simulink model "six_plus_six_AcmsteeringV09_main"  (R2014a)
settings: Solver=FixedStepDiscrete  StartTime=0.0  StopTime=10.0  FixedStep=0.0005  RelTol=1e-3
InitFcn:
  | Veh_Par_wxt
values from neighbouring files (symbols this model uses):
  acc_spdctl = [0 100]    [Veh_Par_wxt.m]
  ag_thr = ecucoder_cal(ag_thr)    [Veh_Par_wxt.m]
  B = 1.8    [Veh_Par_wxt.m]
  bra_em = 100    [Veh_Par_wxt.m]
  bra_pre_gz2 = 100/3    (= 33.3333333333)    [Veh_Par_wxt.m]
  bra_pre_gz34 = 10/3    (= 3.33333333333)    [Veh_Par_wxt.m]
  bra_pre_yd = 10/2    (= 5)    [Veh_Par_wxt.m]
  brakepre_dem_data = [0 1 2 3 4 5 6 7 8 9 10]    [Veh_Par_wxt.m]
  brakeTrq_dem_data = [0 125 251 376 502 627 753 878 1004 1129 1255]    [Veh_Par_wxt.m]
  bratrq_max = 4*1255    (= 5020)    [Veh_Par_wxt.m]
  eff_tran = 0.9    [Veh_Par_wxt.m]
  ESP_switch = ecucoder_cal(ESP_switch)    [Veh_Par_wxt.m]
  G = Mass*g    (= 15696)    [Veh_Par_wxt.m]
  kd1 = ecucoder_cal(kd1)    [Veh_Par_wxt.m]
  kd2 = 0    [Veh_Par_wxt.m]
  ki1 = ecucoder_cal(ki1)    [Veh_Par_wxt.m]
  ki2 = 1    [Veh_Par_wxt.m]
  kp1 = ecucoder_cal(kp1)    [Veh_Par_wxt.m]
  kp2 = 300    [Veh_Par_wxt.m]
  L = L1+L2    (= 2.9)    [Veh_Par_wxt.m]
  premax = 100    [Veh_Par_wxt.m]
  Radius = 0.4572/2    (= 0.2286)    [Veh_Par_wxt.m]
  RC_switch = ecucoder_cal(RC_switch)    [Veh_Par_wxt.m]
  s_opt_yi = 0.15    [Veh_Par_wxt.m]
  s_opt_zhuan = 0.8    [Veh_Par_wxt.m]
  s_opt_zhuan_add = 0.05    [Veh_Par_wxt.m]
  s_opt_zhuan_table = [0.8 0.8 0.3 0.3]    [Veh_Par_wxt.m]
  spd_map_mot = [0 499.85 999.79 1500 2000 2500 3000 3500 4000 4500 4999.8 5999.8]    [Veh_Par_wxt.m]
  spd_spdctl = [0 500]    [Veh_Par_wxt.m]
  speed_thr_park = 5/3.6/Radius*tras_ratio*30/pi    (= 464.143899364)    [Veh_Par_wxt.m]
  TCS_switch = ecucoder_cal(TCS_switch)    [Veh_Par_wxt.m]
  tras_ratio = 8    [Veh_Par_wxt.m]
  trq_map_mot = [70.5 70.012 71.154 65.797 53.917 45.159 38.073 32.685 27.48 17.133 14.949 10.07]    [Veh_Par_wxt.m]
  trqmax_yd = 70.5    [Veh_Par_wxt.m]
  trqmax_zx = 70.5    [Veh_Par_wxt.m]
  trqmaxneg = -70.5    [Veh_Par_wxt.m]
  v_gain = 0.9    [Veh_Par_wxt.m]
  v_table = [0 5 20 100]    [Veh_Par_wxt.m]
  v_thr_park = 5    [Veh_Par_wxt.m]
  zhidong_bianmazhi = [-140000 750000]    [Veh_Par_wxt.m]
  zhidong_down = -140000    [Veh_Par_wxt.m]
  zhidong_up = 750000    [Veh_Par_wxt.m]
  zhidong_youmen = [0 100]    [Veh_Par_wxt.m]
  zhuanxiang_bianmazhi = [-400000 0 400000]    [Veh_Par_wxt.m]
  zhuanxiang_down = -400000    [Veh_Par_wxt.m]
  zhuanxiang_up = 400000    [Veh_Par_wxt.m]
  zhuanxiang_youmen = [-100 0 100]    [Veh_Par_wxt.m]
undefined symbols (not defined in the file or in its folder): ecucoder_acal, guzhang_lf, guzhang_lm, guzhang_lr, guzhang_rf, guzhang_rm, guzhang_rr, myFIS
libraries: simulink x979, ec5744lib x59, fuzblock x2
(part 9 of 26)

== system six_plus_six_AcmsteeringV09_main/Data_input/MCU1_3/MCU1 ==
  input : Inport
  Enable : EnablePort
  Demux : Demux  Outputs=8
  MCU1_ControlTemp_Ad : Sum
  MCU1_ControlTemp_Convert : DataTypeConversion  OutDataTypeStr=uint32
  MCU1_ControlTemp_F : Gain
  MCU1_ControlTemp_L : simulink/Logic and Bit Operations/Bitwise Operator  logicop=AND  UseBitMask=on  BitMask=255  BitMaskRealWorld=Stored Integer
  MCU1_ControlTemp_O : Constant  Value=-40  OutDataTypeStr=single
  MCU1_ControlTemp_S : ArithShift
  MCU1_ControlTemp_Sub : Subsystem
  MCU1_ControlTemp_sat : Saturate  UpperLimit=215  LowerLimit=-40
  MCU1_ControlTempcv : DataTypeConversion
  MCU1_Idc_Ad : Sum
  MCU1_Idc_Convert : DataTypeConversion  OutDataTypeStr=uint32
  MCU1_Idc_F : Gain  Gain=0.1
  MCU1_Idc_L : simulink/Logic and Bit Operations/Bitwise Operator  logicop=AND  UseBitMask=on  BitMask=65535  BitMaskRealWorld=Stored Integer
  MCU1_Idc_O : Constant  Value=-1600  OutDataTypeStr=single
  MCU1_Idc_S : ArithShift
  MCU1_Idc_Sub : Subsystem
  MCU1_Idc_sat : Saturate  UpperLimit=1600  LowerLimit=-1600
  MCU1_Idccv : DataTypeConversion
  MCU1_Idcinput3_Ad : Sum
  MCU1_Idcinput3_C : Constant  Value=256
  MCU1_Idcinput3_P : Product
  MCU1_MotorTemp_Ad : Sum
  MCU1_MotorTemp_Convert : DataTypeConversion  OutDataTypeStr=uint32
  MCU1_MotorTemp_F : Gain
  MCU1_MotorTemp_L : simulink/Logic and Bit Operations/Bitwise Operator  logicop=AND  UseBitMask=on  BitMask=255  BitMaskRealWorld=Stored Integer
  MCU1_MotorTemp_O : Constant  Value=-40  OutDataTypeStr=single
  MCU1_MotorTemp_S : ArithShift
  MCU1_MotorTemp_Sub : Subsystem
  MCU1_MotorTemp_sat : Saturate  UpperLimit=215  LowerLimit=-40
  MCU1_MotorTempcv : DataTypeConversion
  MCU1_PowerFdk_Ad : Sum
  MCU1_PowerFdk_Convert : DataTypeConversion  OutDataTypeStr=uint32
  MCU1_PowerFdk_F : Gain
  MCU1_PowerFdk_L : simulink/Logic and Bit Operations/Bitwise Operator  logicop=AND  UseBitMask=on  BitMask=65535  BitMaskRealWorld=Stored Integer
  MCU1_PowerFdk_O : Constant  Value=0  OutDataTypeStr=single
  MCU1_PowerFdk_S : ArithShift
  MCU1_PowerFdk_Sub : Subsystem
  MCU1_PowerFdk_sat : Saturate  UpperLimit=65535  LowerLimit=0
  MCU1_PowerFdkcv : DataTypeConversion
  MCU1_PowerFdkinput5_Ad : Sum
  MCU1_PowerFdkinput5_C : Constant  Value=256
  MCU1_PowerFdkinput5_P : Product
  MCU1_Udc_Ad : Sum
  MCU1_Udc_Convert : DataTypeConversion  OutDataTypeStr=uint32
  MCU1_Udc_F : Gain  Gain=0.1
  MCU1_Udc_L : simulink/Logic and Bit Operations/Bitwise Operator  logicop=AND  UseBitMask=on  BitMask=65535  BitMaskRealWorld=Stored Integer
  MCU1_Udc_O : Constant  Value=0  OutDataTypeStr=single
  MCU1_Udc_S : ArithShift
  MCU1_Udc_Sub : Subsystem
  MCU1_Udc_sat : Saturate  UpperLimit=1000  LowerLimit=0
  MCU1_Udccv : DataTypeConversion
  MCU1_Udcinput1_Ad : Sum
  MCU1_Udcinput1_C : Constant  Value=256
  MCU1_Udcinput1_P : Product
  MCU1_ControlTemp_Out : Outport
  MCU1_MotorTemp_Out : Outport  Port=2
  MCU1_PowerFdk_Out : Outport  Port=3
  MCU1_Idc_Out : Outport  Port=4
  MCU1_Udc_Out : Outport  Port=5
  wires:
  MCU1_ControlTemp_F/1 -> MCU1_ControlTemp_Ad/1
  MCU1_ControlTemp_O/1 -> MCU1_ControlTemp_Ad/2
  MCU1_ControlTemp_Ad/1 -> MCU1_ControlTemp_sat/1
  MCU1_ControlTemp_sat/1 -> MCU1_ControlTemp_Out/1
  Demux/8 -> MCU1_ControlTemp_Sub/1(In1)
  MCU1_ControlTemp_Sub/1(Out1) -> MCU1_ControlTemp_Convert/1
  MCU1_ControlTemp_Convert/1 -> MCU1_ControlTemp_L/1
  MCU1_ControlTemp_L/1 -> MCU1_ControlTemp_S/1
  MCU1_ControlTemp_S/1 -> MCU1_ControlTempcv/1
  MCU1_ControlTempcv/1 -> MCU1_ControlTemp_F/1
  MCU1_MotorTemp_F/1 -> MCU1_MotorTemp_Ad/1
  MCU1_MotorTemp_O/1 -> MCU1_MotorTemp_Ad/2
  MCU1_MotorTemp_Ad/1 -> MCU1_MotorTemp_sat/1
  MCU1_MotorTemp_sat/1 -> MCU1_MotorTemp_Out/1
  Demux/7 -> MCU1_MotorTemp_Sub/1(In1)
  MCU1_MotorTemp_Sub/1(Out1) -> MCU1_MotorTemp_Convert/1
  MCU1_MotorTemp_Convert/1 -> MCU1_MotorTemp_L/1
  MCU1_MotorTemp_L/1 -> MCU1_MotorTemp_S/1
  MCU1_MotorTemp_S/1 -> MCU1_MotorTempcv/1
  MCU1_MotorTempcv/1 -> MCU1_MotorTemp_F/1
  MCU1_PowerFdk_F/1 -> MCU1_PowerFdk_Ad/1
  MCU1_PowerFdk_O/1 -> MCU1_PowerFdk_Ad/2
  MCU1_PowerFdk_Ad/1 -> MCU1_PowerFdk_sat/1
  MCU1_PowerFdk_sat/1 -> MCU1_PowerFdk_Out/1
  Demux/5 -> MCU1_PowerFdkinput5_P/1
  MCU1_PowerFdkinput5_C/1 -> MCU1_PowerFdkinput5_P/2
  MCU1_PowerFdkinput5_P/1 -> MCU1_PowerFdkinput5_Ad/1
  Demux/6 -> MCU1_PowerFdkinput5_Ad/2
  MCU1_PowerFdkinput5_Ad/1 -> MCU1_PowerFdk_Sub/1(In1)
  MCU1_PowerFdk_Sub/1(Out1) -> MCU1_PowerFdk_Convert/1
  MCU1_PowerFdk_Convert/1 -> MCU1_PowerFdk_L/1
  MCU1_PowerFdk_L/1 -> MCU1_PowerFdk_S/1
  MCU1_PowerFdk_S/1 -> MCU1_PowerFdkcv/1
  MCU1_PowerFdkcv/1 -> MCU1_PowerFdk_F/1
  MCU1_Idc_F/1 -> MCU1_Idc_Ad/1
  MCU1_Idc_O/1 -> MCU1_Idc_Ad/2
  MCU1_Idc_Ad/1 -> MCU1_Idc_sat/1
  MCU1_Idc_sat/1 -> MCU1_Idc_Out/1
  Demux/3 -> MCU1_Idcinput3_P/1
  MCU1_Idcinput3_C/1 -> MCU1_Idcinput3_P/2
  MCU1_Idcinput3_P/1 -> MCU1_Idcinput3_Ad/1
  Demux/4 -> MCU1_Idcinput3_Ad/2
  MCU1_Idcinput3_Ad/1 -> MCU1_Idc_Sub/1(In1)
  MCU1_Idc_Sub/1(Out1) -> MCU1_Idc_Convert/1
  MCU1_Idc_Convert/1 -> MCU1_Idc_L/1
  MCU1_Idc_L/1 -> MCU1_Idc_S/1
  MCU1_Idc_S/1 -> MCU1_Idccv/1
  MCU1_Idccv/1 -> MCU1_Idc_F/1
  MCU1_Udc_F/1 -> MCU1_Udc_Ad/1
  MCU1_Udc_O/1 -> MCU1_Udc_Ad/2
  MCU1_Udc_Ad/1 -> MCU1_Udc_sat/1
  MCU1_Udc_sat/1 -> MCU1_Udc_Out/1
  Demux/1 -> MCU1_Udcinput1_P/1
  MCU1_Udcinput1_C/1 -> MCU1_Udcinput1_P/2
  MCU1_Udcinput1_P/1 -> MCU1_Udcinput1_Ad/1
  Demux/2 -> MCU1_Udcinput1_Ad/2
  MCU1_Udcinput1_Ad/1 -> MCU1_Udc_Sub/1(In1)
  MCU1_Udc_Sub/1(Out1) -> MCU1_Udc_Convert/1
  MCU1_Udc_Convert/1 -> MCU1_Udc_L/1
  MCU1_Udc_L/1 -> MCU1_Udc_S/1
  MCU1_Udc_S/1 -> MCU1_Udccv/1
  MCU1_Udccv/1 -> MCU1_Udc_F/1
  input/1 -> Demux/1

== system six_plus_six_AcmsteeringV09_main/Data_input/MCU1_4/MCU1 ==
  input : Inport
  Enable : EnablePort
  Demux : Demux  Outputs=8
  MCU1_ControlTemp_Ad : Sum
  MCU1_ControlTemp_Convert : DataTypeConversion  OutDataTypeStr=uint32
  MCU1_ControlTemp_F : Gain
  MCU1_ControlTemp_L : simulink/Logic and Bit Operations/Bitwise Operator  logicop=AND  UseBitMask=on  BitMask=255  BitMaskRealWorld=Stored Integer
  MCU1_ControlTemp_O : Constant  Value=-40  OutDataTypeStr=single
  MCU1_ControlTemp_S : ArithShift
  MCU1_ControlTemp_Sub : Subsystem
  MCU1_ControlTemp_sat : Saturate  UpperLimit=215  LowerLimit=-40
  MCU1_ControlTempcv : DataTypeConversion
  MCU1_Idc_Ad : Sum
  MCU1_Idc_Convert : DataTypeConversion  OutDataTypeStr=uint32
  MCU1_Idc_F : Gain  Gain=0.1
  MCU1_Idc_L : simulink/Logic and Bit Operations/Bitwise Operator  logicop=AND  UseBitMask=on  BitMask=65535  BitMaskRealWorld=Stored Integer
  MCU1_Idc_O : Constant  Value=-1600  OutDataTypeStr=single
  MCU1_Idc_S : ArithShift
  MCU1_Idc_Sub : Subsystem
  MCU1_Idc_sat : Saturate  UpperLimit=1600  LowerLimit=-1600
  MCU1_Idccv : DataTypeConversion
  MCU1_Idcinput3_Ad : Sum
  MCU1_Idcinput3_C : Constant  Value=256
  MCU1_Idcinput3_P : Product
  MCU1_MotorTemp_Ad : Sum
  MCU1_MotorTemp_Convert : DataTypeConversion  OutDataTypeStr=uint32
  MCU1_MotorTemp_F : Gain
  MCU1_MotorTemp_L : simulink/Logic and Bit Operations/Bitwise Operator  logicop=AND  UseBitMask=on  BitMask=255  BitMaskRealWorld=Stored Integer
  MCU1_MotorTemp_O : Constant  Value=-40  OutDataTypeStr=single
  MCU1_MotorTemp_S : ArithShift
  MCU1_MotorTemp_Sub : Subsystem
  MCU1_MotorTemp_sat : Saturate  UpperLimit=215  LowerLimit=-40
  MCU1_MotorTempcv : DataTypeConversion
  MCU1_PowerFdk_Ad : Sum
  MCU1_PowerFdk_Convert : DataTypeConversion  OutDataTypeStr=uint32
  MCU1_PowerFdk_F : Gain
  MCU1_PowerFdk_L : simulink/Logic and Bit Operations/Bitwise Operator  logicop=AND  UseBitMask=on  BitMask=65535  BitMaskRealWorld=Stored Integer
  MCU1_PowerFdk_O : Constant  Value=0  OutDataTypeStr=single
  MCU1_PowerFdk_S : ArithShift
  MCU1_PowerFdk_Sub : Subsystem
  MCU1_PowerFdk_sat : Saturate  UpperLimit=65535  LowerLimit=0
  MCU1_PowerFdkcv : DataTypeConversion
  MCU1_PowerFdkinput5_Ad : Sum
  MCU1_PowerFdkinput5_C : Constant  Value=256
  MCU1_PowerFdkinput5_P : Product
  MCU1_Udc_Ad : Sum
  MCU1_Udc_Convert : DataTypeConversion  OutDataTypeStr=uint32
  MCU1_Udc_F : Gain  Gain=0.1
  MCU1_Udc_L : simulink/Logic and Bit Operations/Bitwise Operator  logicop=AND  UseBitMask=on  BitMask=65535  BitMaskRealWorld=Stored Integer
  MCU1_Udc_O : Constant  Value=0  OutDataTypeStr=single
  MCU1_Udc_S : ArithShift
  MCU1_Udc_Sub : Subsystem
  MCU1_Udc_sat : Saturate  UpperLimit=1000  LowerLimit=0
  MCU1_Udccv : DataTypeConversion
  MCU1_Udcinput1_Ad : Sum
  MCU1_Udcinput1_C : Constant  Value=256
  MCU1_Udcinput1_P : Product
  MCU1_ControlTemp_Out : Outport
  MCU1_MotorTemp_Out : Outport  Port=2
  MCU1_PowerFdk_Out : Outport  Port=3
  MCU1_Idc_Out : Outport  Port=4
  MCU1_Udc_Out : Outport  Port=5
  wires:
  MCU1_ControlTemp_F/1 -> MCU1_ControlTemp_Ad/1
  MCU1_ControlTemp_O/1 -> MCU1_ControlTemp_Ad/2
  MCU1_ControlTemp_Ad/1 -> MCU1_ControlTemp_sat/1
  MCU1_ControlTemp_sat/1 -> MCU1_ControlTemp_Out/1
  Demux/8 -> MCU1_ControlTemp_Sub/1(In1)
  MCU1_ControlTemp_Sub/1(Out1) -> MCU1_ControlTemp_Convert/1
  MCU1_ControlTemp_Convert/1 -> MCU1_ControlTemp_L/1
  MCU1_ControlTemp_L/1 -> MCU1_ControlTemp_S/1
  MCU1_ControlTemp_S/1 -> MCU1_ControlTempcv/1
  MCU1_ControlTempcv/1 -> MCU1_ControlTemp_F/1
  MCU1_MotorTemp_F/1 -> MCU1_MotorTemp_Ad/1
  MCU1_MotorTemp_O/1 -> MCU1_MotorTemp_Ad/2
  MCU1_MotorTemp_Ad/1 -> MCU1_MotorTemp_sat/1
  MCU1_MotorTemp_sat/1 -> MCU1_MotorTemp_Out/1
  Demux/7 -> MCU1_MotorTemp_Sub/1(In1)
  MCU1_MotorTemp_Sub/1(Out1) -> MCU1_MotorTemp_Convert/1
  MCU1_MotorTemp_Convert/1 -> MCU1_MotorTemp_L/1
  MCU1_MotorTemp_L/1 -> MCU1_MotorTemp_S/1
  MCU1_MotorTemp_S/1 -> MCU1_MotorTempcv/1
  MCU1_MotorTempcv/1 -> MCU1_MotorTemp_F/1
  MCU1_PowerFdk_F/1 -> MCU1_PowerFdk_Ad/1
  MCU1_PowerFdk_O/1 -> MCU1_PowerFdk_Ad/2
  MCU1_PowerFdk_Ad/1 -> MCU1_PowerFdk_sat/1
  MCU1_PowerFdk_sat/1 -> MCU1_PowerFdk_Out/1
  Demux/5 -> MCU1_PowerFdkinput5_P/1
  MCU1_PowerFdkinput5_C/1 -> MCU1_PowerFdkinput5_P/2
  MCU1_PowerFdkinput5_P/1 -> MCU1_PowerFdkinput5_Ad/1
  Demux/6 -> MCU1_PowerFdkinput5_Ad/2
  MCU1_PowerFdkinput5_Ad/1 -> MCU1_PowerFdk_Sub/1(In1)
  MCU1_PowerFdk_Sub/1(Out1) -> MCU1_PowerFdk_Convert/1
  MCU1_PowerFdk_Convert/1 -> MCU1_PowerFdk_L/1
  MCU1_PowerFdk_L/1 -> MCU1_PowerFdk_S/1
  MCU1_PowerFdk_S/1 -> MCU1_PowerFdkcv/1
  MCU1_PowerFdkcv/1 -> MCU1_PowerFdk_F/1
  MCU1_Idc_F/1 -> MCU1_Idc_Ad/1
  MCU1_Idc_O/1 -> MCU1_Idc_Ad/2
  MCU1_Idc_Ad/1 -> MCU1_Idc_sat/1
  MCU1_Idc_sat/1 -> MCU1_Idc_Out/1
  Demux/3 -> MCU1_Idcinput3_P/1
  MCU1_Idcinput3_C/1 -> MCU1_Idcinput3_P/2
  MCU1_Idcinput3_P/1 -> MCU1_Idcinput3_Ad/1
  Demux/4 -> MCU1_Idcinput3_Ad/2
  MCU1_Idcinput3_Ad/1 -> MCU1_Idc_Sub/1(In1)
  MCU1_Idc_Sub/1(Out1) -> MCU1_Idc_Convert/1
  MCU1_Idc_Convert/1 -> MCU1_Idc_L/1
  MCU1_Idc_L/1 -> MCU1_Idc_S/1
  MCU1_Idc_S/1 -> MCU1_Idccv/1
  MCU1_Idccv/1 -> MCU1_Idc_F/1
  MCU1_Udc_F/1 -> MCU1_Udc_Ad/1
  MCU1_Udc_O/1 -> MCU1_Udc_Ad/2
  MCU1_Udc_Ad/1 -> MCU1_Udc_sat/1
  MCU1_Udc_sat/1 -> MCU1_Udc_Out/1
  Demux/1 -> MCU1_Udcinput1_P/1
  MCU1_Udcinput1_C/1 -> MCU1_Udcinput1_P/2
  MCU1_Udcinput1_P/1 -> MCU1_Udcinput1_Ad/1
  Demux/2 -> MCU1_Udcinput1_Ad/2
  MCU1_Udcinput1_Ad/1 -> MCU1_Udc_Sub/1(In1)
  MCU1_Udc_Sub/1(Out1) -> MCU1_Udc_Convert/1
  MCU1_Udc_Convert/1 -> MCU1_Udc_L/1
  MCU1_Udc_L/1 -> MCU1_Udc_S/1
  MCU1_Udc_S/1 -> MCU1_Udccv/1
  MCU1_Udccv/1 -> MCU1_Udc_F/1
  input/1 -> Demux/1

== system six_plus_six_AcmsteeringV09_main/Data_input/MCU1_5/MCU1 ==
  input : Inport
  Enable : EnablePort
  Demux : Demux  Outputs=8
  MCU1_ControlTemp_Ad : Sum
  MCU1_ControlTemp_Convert : DataTypeConversion  OutDataTypeStr=uint32
  MCU1_ControlTemp_F : Gain
  MCU1_ControlTemp_L : simulink/Logic and Bit Operations/Bitwise Operator  logicop=AND  UseBitMask=on  BitMask=255  BitMaskRealWorld=Stored Integer
  MCU1_ControlTemp_O : Constant  Value=-40  OutDataTypeStr=single
  MCU1_ControlTemp_S : ArithShift
  MCU1_ControlTemp_Sub : Subsystem
  MCU1_ControlTemp_sat : Saturate  UpperLimit=215  LowerLimit=-40
  MCU1_ControlTempcv : DataTypeConversion
  MCU1_Idc_Ad : Sum
  MCU1_Idc_Convert : DataTypeConversion  OutDataTypeStr=uint32
  MCU1_Idc_F : Gain  Gain=0.1
  MCU1_Idc_L : simulink/Logic and Bit Operations/Bitwise Operator  logicop=AND  UseBitMask=on  BitMask=65535  BitMaskRealWorld=Stored Integer
  MCU1_Idc_O : Constant  Value=-1600  OutDataTypeStr=single
  MCU1_Idc_S : ArithShift
  MCU1_Idc_Sub : Subsystem
  MCU1_Idc_sat : Saturate  UpperLimit=1600  LowerLimit=-1600
  MCU1_Idccv : DataTypeConversion
  MCU1_Idcinput3_Ad : Sum
  MCU1_Idcinput3_C : Constant  Value=256
  MCU1_Idcinput3_P : Product
  MCU1_MotorTemp_Ad : Sum
  MCU1_MotorTemp_Convert : DataTypeConversion  OutDataTypeStr=uint32
  MCU1_MotorTemp_F : Gain
  MCU1_MotorTemp_L : simulink/Logic and Bit Operations/Bitwise Operator  logicop=AND  UseBitMask=on  BitMask=255  BitMaskRealWorld=Stored Integer
  MCU1_MotorTemp_O : Constant  Value=-40  OutDataTypeStr=single
  MCU1_MotorTemp_S : ArithShift
  MCU1_MotorTemp_Sub : Subsystem
  MCU1_MotorTemp_sat : Saturate  UpperLimit=215  LowerLimit=-40
  MCU1_MotorTempcv : DataTypeConversion
  MCU1_PowerFdk_Ad : Sum
  MCU1_PowerFdk_Convert : DataTypeConversion  OutDataTypeStr=uint32
  MCU1_PowerFdk_F : Gain
  MCU1_PowerFdk_L : simulink/Logic and Bit Operations/Bitwise Operator  logicop=AND  UseBitMask=on  BitMask=65535  BitMaskRealWorld=Stored Integer
  MCU1_PowerFdk_O : Constant  Value=0  OutDataTypeStr=single
  MCU1_PowerFdk_S : ArithShift
  MCU1_PowerFdk_Sub : Subsystem
  MCU1_PowerFdk_sat : Saturate  UpperLimit=65535  LowerLimit=0
  MCU1_PowerFdkcv : DataTypeConversion
  MCU1_PowerFdkinput5_Ad : Sum
  MCU1_PowerFdkinput5_C : Constant  Value=256
  MCU1_PowerFdkinput5_P : Product
  MCU1_Udc_Ad : Sum
  MCU1_Udc_Convert : DataTypeConversion  OutDataTypeStr=uint32
  MCU1_Udc_F : Gain  Gain=0.1
  MCU1_Udc_L : simulink/Logic and Bit Operations/Bitwise Operator  logicop=AND  UseBitMask=on  BitMask=65535  BitMaskRealWorld=Stored Integer
  MCU1_Udc_O : Constant  Value=0  OutDataTypeStr=single
  MCU1_Udc_S : ArithShift
  MCU1_Udc_Sub : Subsystem
  MCU1_Udc_sat : Saturate  UpperLimit=1000  LowerLimit=0
  MCU1_Udccv : DataTypeConversion
  MCU1_Udcinput1_Ad : Sum
  MCU1_Udcinput1_C : Constant  Value=256
  MCU1_Udcinput1_P : Product
  MCU1_ControlTemp_Out : Outport
  MCU1_MotorTemp_Out : Outport  Port=2
  MCU1_PowerFdk_Out : Outport  Port=3
  MCU1_Idc_Out : Outport  Port=4
  MCU1_Udc_Out : Outport  Port=5
  wires:
  MCU1_ControlTemp_F/1 -> MCU1_ControlTemp_Ad/1
  MCU1_ControlTemp_O/1 -> MCU1_ControlTemp_Ad/2
  MCU1_ControlTemp_Ad/1 -> MCU1_ControlTemp_sat/1
  MCU1_ControlTemp_sat/1 -> MCU1_ControlTemp_Out/1
  Demux/8 -> MCU1_ControlTemp_Sub/1(In1)
  MCU1_ControlTemp_Sub/1(Out1) -> MCU1_ControlTemp_Convert/1
  MCU1_ControlTemp_Convert/1 -> MCU1_ControlTemp_L/1
  MCU1_ControlTemp_L/1 -> MCU1_ControlTemp_S/1
  MCU1_ControlTemp_S/1 -> MCU1_ControlTempcv/1
  MCU1_ControlTempcv/1 -> MCU1_ControlTemp_F/1
  MCU1_MotorTemp_F/1 -> MCU1_MotorTemp_Ad/1
  MCU1_MotorTemp_O/1 -> MCU1_MotorTemp_Ad/2
  MCU1_MotorTemp_Ad/1 -> MCU1_MotorTemp_sat/1
  MCU1_MotorTemp_sat/1 -> MCU1_MotorTemp_Out/1
  Demux/7 -> MCU1_MotorTemp_Sub/1(In1)
  MCU1_MotorTemp_Sub/1(Out1) -> MCU1_MotorTemp_Convert/1
  MCU1_MotorTemp_Convert/1 -> MCU1_MotorTemp_L/1
  MCU1_MotorTemp_L/1 -> MCU1_MotorTemp_S/1
  MCU1_MotorTemp_S/1 -> MCU1_MotorTempcv/1
  MCU1_MotorTempcv/1 -> MCU1_MotorTemp_F/1
  MCU1_PowerFdk_F/1 -> MCU1_PowerFdk_Ad/1
  MCU1_PowerFdk_O/1 -> MCU1_PowerFdk_Ad/2
  MCU1_PowerFdk_Ad/1 -> MCU1_PowerFdk_sat/1
  MCU1_PowerFdk_sat/1 -> MCU1_PowerFdk_Out/1
  Demux/5 -> MCU1_PowerFdkinput5_P/1
  MCU1_PowerFdkinput5_C/1 -> MCU1_PowerFdkinput5_P/2
  MCU1_PowerFdkinput5_P/1 -> MCU1_PowerFdkinput5_Ad/1
  Demux/6 -> MCU1_PowerFdkinput5_Ad/2
  MCU1_PowerFdkinput5_Ad/1 -> MCU1_PowerFdk_Sub/1(In1)
  MCU1_PowerFdk_Sub/1(Out1) -> MCU1_PowerFdk_Convert/1
  MCU1_PowerFdk_Convert/1 -> MCU1_PowerFdk_L/1
  MCU1_PowerFdk_L/1 -> MCU1_PowerFdk_S/1
  MCU1_PowerFdk_S/1 -> MCU1_PowerFdkcv/1
  MCU1_PowerFdkcv/1 -> MCU1_PowerFdk_F/1
  MCU1_Idc_F/1 -> MCU1_Idc_Ad/1
  MCU1_Idc_O/1 -> MCU1_Idc_Ad/2
  MCU1_Idc_Ad/1 -> MCU1_Idc_sat/1
  MCU1_Idc_sat/1 -> MCU1_Idc_Out/1
  Demux/3 -> MCU1_Idcinput3_P/1
  MCU1_Idcinput3_C/1 -> MCU1_Idcinput3_P/2
  MCU1_Idcinput3_P/1 -> MCU1_Idcinput3_Ad/1
  Demux/4 -> MCU1_Idcinput3_Ad/2
  MCU1_Idcinput3_Ad/1 -> MCU1_Idc_Sub/1(In1)
  MCU1_Idc_Sub/1(Out1) -> MCU1_Idc_Convert/1
  MCU1_Idc_Convert/1 -> MCU1_Idc_L/1
  MCU1_Idc_L/1 -> MCU1_Idc_S/1
  MCU1_Idc_S/1 -> MCU1_Idccv/1
  MCU1_Idccv/1 -> MCU1_Idc_F/1
  MCU1_Udc_F/1 -> MCU1_Udc_Ad/1
  MCU1_Udc_O/1 -> MCU1_Udc_Ad/2
  MCU1_Udc_Ad/1 -> MCU1_Udc_sat/1
  MCU1_Udc_sat/1 -> MCU1_Udc_Out/1
  Demux/1 -> MCU1_Udcinput1_P/1
  MCU1_Udcinput1_C/1 -> MCU1_Udcinput1_P/2
  MCU1_Udcinput1_P/1 -> MCU1_Udcinput1_Ad/1
  Demux/2 -> MCU1_Udcinput1_Ad/2
  MCU1_Udcinput1_Ad/1 -> MCU1_Udc_Sub/1(In1)
  MCU1_Udc_Sub/1(Out1) -> MCU1_Udc_Convert/1
  MCU1_Udc_Convert/1 -> MCU1_Udc_L/1
  MCU1_Udc_L/1 -> MCU1_Udc_S/1
  MCU1_Udc_S/1 -> MCU1_Udccv/1
  MCU1_Udccv/1 -> MCU1_Udc_F/1
  input/1 -> Demux/1

== matlab function six_plus_six_AcmsteeringV09_main/MainControl/mode_control/neutral/neutral/HeartBeat3 ==
  data: life_pre input; life output
function life = fcn(life_pre)
%#codegen
life=single(life_pre+1);
if life>255
    life=single(0);
end
end

== matlab function six_plus_six_AcmsteeringV09_main/MainControl/mode_control/backward/backward/Brake/HeartBeat5 ==
  data: life_pre input; life output
function life = fcn(life_pre)
%#codegen
life=single(life_pre+1);
if life>255
    life=single(0);
end
end

== matlab function six_plus_six_AcmsteeringV09_main/MainControl/mode_control/backward/backward/Drive/目标转向力矩确定模块/MATLAB Function2 ==
  data: umax input; delta_Tsteer_max output; G input; L input; B input; Radius input; Rturn_min_xy input
function delta_Tsteer_max = fcn(umax,G,L,B,Radius,Rturn_min_xy)
%#codegen

    delta_Fsteer_max=single(umax/(0.925+0.15*(Rturn_min_xy/B))*G*L/(2*B));
    delta_Tsteer_max=single(delta_Fsteer_max*Radius);
    
end

== matlab function six_plus_six_AcmsteeringV09_main/MainControl/mode_control/forward/forward/MATLAB Function ==
  data: acc_dem input; y output; brake_dem input; HAC input
function y = fcn(acc_dem,brake_dem,HAC)
%#codegen
if HAC==1
    if acc_dem>0
        y=int8(0);
    else
        y=int8(1);
    end
else
    if brake_dem==0
        y=int8(0);
    else
        y=int8(1);
    end
end
end

== matlab function six_plus_six_AcmsteeringV09_main/MainControl/mode_control/backward/backward/Drive/驱动防滑控制TCS/直行TCS/直行/HeartBeat5 ==
  data: life_pre input; life output
function life = fcn(life_pre)
%#codegen
life=single(life_pre+1);
if life>255
    life=single(0);
end
end

== matlab function six_plus_six_AcmsteeringV09_main/MainControl/mode_control/center_steer/center_steer/HeartBeat1 ==
  data: life_pre input; life output
function life = fcn(life_pre)
%#codegen
life=single(life_pre+1);
if life>255
    life=single(0);
end
end

== matlab function six_plus_six_AcmsteeringV09_main/MainControl/mode_control/emergency_stop/emergency_stop/HeartBeat4 ==
  data: life_pre input; life output
function life = fcn(life_pre)
%#codegen
life=single(life_pre+1);
if life>255
    life=single(0);
end
end

== matlab function six_plus_six_AcmsteeringV09_main/Data_input/2/Enabled Subsystem/MATLAB Function1 ==
  data: current_in input; current_out output
function current_out = motec_current(current_in)
    if current_in>32768
        current_out=current_in-65535;
    else
        current_out=current_in;
    end
end

== matlab function six_plus_six_AcmsteeringV09_main/MainControl/mode_control/backward/backward/Drive/驱动防滑控制TCS/直行TCS/直行/MATLAB Function4 ==
  data: s_act_lm input; flag_lm output; s_opt_zhuan input; s_opt_zhuan_add input; flag_lm_pre input int8
function flag_lm = fcn(s_act_lm,s_opt_zhuan,s_opt_zhuan_add,flag_lm_pre)
%#codegen
if s_act_lm>s_opt_zhuan+s_opt_zhuan_add
    flag_lm=int8(1);
elseif s_act_lm<s_opt_zhuan
    flag_lm =int8(0);
else
    flag_lm=int8(flag_lm_pre);
end
end

== matlab function six_plus_six_AcmsteeringV09_main/Data_input/6/Enabled
Subsystem/MATLAB Function ==
  data: data1 input; y output; data2 input; data3 input; data4 input
function y = fcn(data1,data2,data3,data4)
%#codegen
y1=data4*256^3+data3*256^2+data2*256+data1;
y=typecast(uint32(y1),'single');
end
% y = u;

== matlab function six_plus_six_AcmsteeringV09_main/Data_input/9/Enabled Subsystem/MATLAB Function ==
  data: data1 input; y output; data2 input; data3 input; data4 input
function y = fcn(data1,data2,data3,data4)
%#codegen
y1=data4*256^3+data3*256^2+data2*256+data1;
% y=typecast(uint32(y1),'single');
y=single(y1*10^-7);
end
% y = u;

== matlab function six_plus_six_AcmsteeringV09_main/MainControl/mode_control/backward/backward/Drive/容错控制/MATLAB Function5 ==
  data: RC_switch input; guzhang_lf1 output; guzhang_lm1 output; guzhang_lf input; guzhang_lm input; guzhang_lr input; guzhang_lr1 output; guzhang_rf input; guzhang_rm input; guzhang_rr input; guzhang_rf1 output; guzhang_rm1 output; guzhang_rr1 output
 function [guzhang_lf1,guzhang_lm1,guzhang_lr1,guzhang_rf1,guzhang_rm1,guzhang_rr1] = fcn(RC_switch,guzhang_lf,guzhang_lm,guzhang_lr,guzhang_rf,guzhang_rm,guzhang_rr)
%#codegen
if RC_switch==0
    guzhang_lf1=single(0);
    guzhang_lm1=single(0);
    guzhang_lr1=single(0);
    guzhang_rf1=single(0);
    guzhang_rm1=single(0);
    guzhang_rr1=single(0);
else
    guzhang_lf1=single(guzhang_lf);
    guzhang_lm1=single(guzhang_lm);
    guzhang_lr1=single(guzhang_lr);
    guzhang_rf1=single(guzhang_rf);
    guzhang_rm1=single(guzhang_rm);
    guzhang_rr1=single(guzhang_rr);
end
end

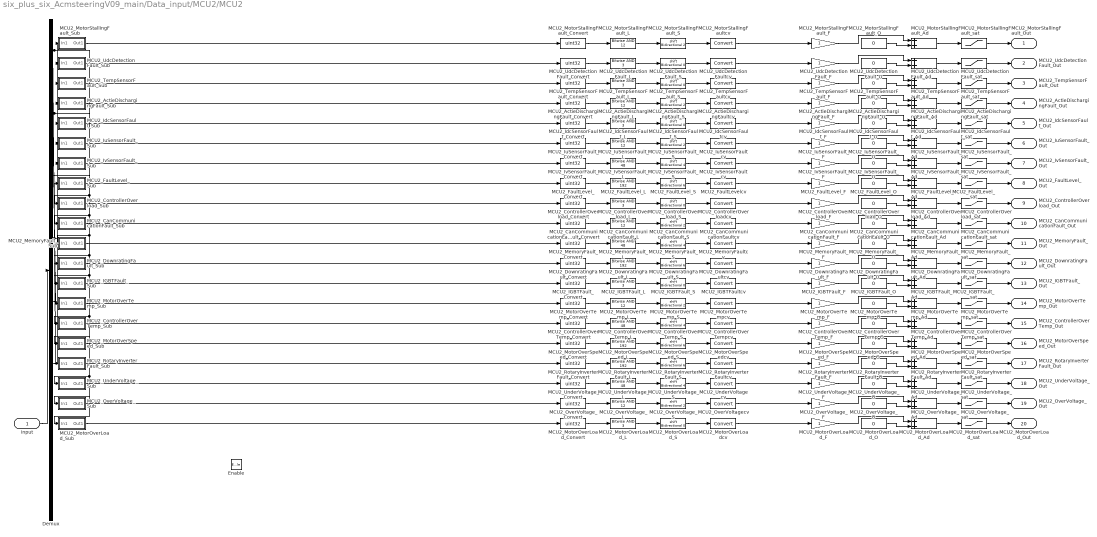
== system six_plus_six_AcmsteeringV09_main/Data_input/MCU2/MCU2 ==
  input : Inport
  Enable : EnablePort
  Demux : Demux  Outputs=8
  MCU2_ActieDischargingFault_Ad : Sum
  MCU2_ActieDischargingFault_Convert : DataTypeConversion  OutDataTypeStr=uint32
  MCU2_ActieDischargingFault_F : Gain
  MCU2_ActieDischargingFault_L : simulink/Logic and Bit Operations/Bitwise Operator  logicop=AND  UseBitMask=on  BitMask=12  BitMaskRealWorld=Stored Integer
  MCU2_ActieDischargingFault_O : Constant  Value=0  OutDataTypeStr=single
  MCU2_ActieDischargingFault_S : ArithShift  BitShiftNumber=2
  MCU2_ActieDischargingFault_Sub : Subsystem
  MCU2_ActieDischargingFault_sat : Saturate  UpperLimit=3  LowerLimit=0
  MCU2_ActieDischargingFaultcv : DataTypeConversion
  MCU2_CanCommunicationFault_Ad : Sum
  MCU2_CanCommunicationFault_Convert : DataTypeConversion  OutDataTypeStr=uint32
  MCU2_CanCommunicationFault_F : Gain
  MCU2_CanCommunicationFault_L : simulink/Logic and Bit Operations/Bitwise Operator  logicop=AND  UseBitMask=on  BitMask=12  BitMaskRealWorld=Stored Integer
  MCU2_CanCommunicationFault_O : Constant  Value=0  OutDataTypeStr=single
  MCU2_CanCommunicationFault_S : ArithShift  BitShiftNumber=2
  MCU2_CanCommunicationFault_Sub : Subsystem
  MCU2_CanCommunicationFault_sat : Saturate  UpperLimit=3  LowerLimit=0
  MCU2_CanCommunicationFaultcv : DataTypeConversion
  MCU2_ControllerOverTemp_Ad : Sum
  MCU2_ControllerOverTemp_Convert : DataTypeConversion  OutDataTypeStr=uint32
  MCU2_ControllerOverTemp_F : Gain
  MCU2_ControllerOverTemp_L : simulink/Logic and Bit Operations/Bitwise Operator  logicop=AND  UseBitMask=on  BitMask=48  BitMaskRealWorld=Stored Integer
  MCU2_ControllerOverTemp_O : Constant  Value=0  OutDataTypeStr=single
  MCU2_ControllerOverTemp_S : ArithShift  BitShiftNumber=4
  MCU2_ControllerOverTemp_Sub : Subsystem
  MCU2_ControllerOverTemp_sat : Saturate  UpperLimit=3  LowerLimit=0
  MCU2_ControllerOverTempcv : DataTypeConversion
  MCU2_ControllerOverload_Ad : Sum
  MCU2_ControllerOverload_Convert : DataTypeConversion  OutDataTypeStr=uint32
  MCU2_ControllerOverload_F : Gain
  MCU2_ControllerOverload_L : simulink/Logic and Bit Operations/Bitwise Operator  logicop=AND  UseBitMask=on  BitMask=3  BitMaskRealWorld=Stored Integer
  MCU2_ControllerOverload_O : Constant  Value=0  OutDataTypeStr=single
  MCU2_ControllerOverload_S : ArithShift
  MCU2_ControllerOverload_Sub : Subsystem
  MCU2_ControllerOverload_sat : Saturate  UpperLimit=3  LowerLimit=0
  MCU2_ControllerOverloadcv : DataTypeConversion
  MCU2_DownratingFault_Ad : Sum
  MCU2_DownratingFault_Convert : DataTypeConversion  OutDataTypeStr=uint32
  MCU2_DownratingFault_F : Gain
  MCU2_DownratingFault_L : simulink/Logic and Bit Operations/Bitwise Operator  logicop=AND  UseBitMask=on  BitMask=192  BitMaskRealWorld=Stored Integer
  MCU2_DownratingFault_O : Constant  Value=0  OutDataTypeStr=single
  MCU2_DownratingFault_S : ArithShift  BitShiftNumber=6
  MCU2_DownratingFault_Sub : Subsystem
  MCU2_DownratingFault_sat : Saturate  UpperLimit=3  LowerLimit=0
  MCU2_DownratingFaultcv : DataTypeConversion
  MCU2_FaultLevel_Ad : Sum
  MCU2_FaultLevel_Convert : DataTypeConversion  OutDataTypeStr=uint32
  MCU2_FaultLevel_F : Gain
  MCU2_FaultLevel_L : simulink/Logic and Bit Operations/Bitwise Operator  logicop=AND  UseBitMask=on  BitMask=192  BitMaskRealWorld=Stored Integer
  MCU2_FaultLevel_O : Constant  Value=0  OutDataTypeStr=single
  MCU2_FaultLevel_S : ArithShift  BitShiftNumber=6
  MCU2_FaultLevel_Sub : Subsystem
  MCU2_FaultLevel_sat : Saturate  UpperLimit=3  LowerLimit=0
  MCU2_FaultLevelcv : DataTypeConversion
  MCU2_IGBTFault_Ad : Sum
  MCU2_IGBTFault_Convert : DataTypeConversion  OutDataTypeStr=uint32
  MCU2_IGBTFault_F : Gain
  MCU2_IGBTFault_L : simulink/Logic and Bit Operations/Bitwise Operator  logicop=AND  UseBitMask=on  BitMask=3  BitMaskRealWorld=Stored Integer
  MCU2_IGBTFault_O : Constant  Value=0  OutDataTypeStr=single
  MCU2_IGBTFault_S : ArithShift
  MCU2_IGBTFault_Sub : Subsystem
  MCU2_IGBTFault_sat : Saturate  UpperLimit=3  LowerLimit=0
  MCU2_IGBTFaultcv : DataTypeConversion
  MCU2_IdcSensorFault_Ad : Sum
  MCU2_IdcSensorFault_Convert : DataTypeConversion  OutDataTypeStr=uint32
  MCU2_IdcSensorFault_F : Gain
  MCU2_IdcSensorFault_L : simulink/Logic and Bit Operations/Bitwise Operator  logicop=AND  UseBitMask=on  BitMask=3  BitMaskRealWorld=Stored Integer
  MCU2_IdcSensorFault_O : Constant  Value=0  OutDataTypeStr=single
  MCU2_IdcSensorFault_S : ArithShift
  MCU2_IdcSensorFault_Sub : Subsystem
  MCU2_IdcSensorFault_sat : Saturate  UpperLimit=3  LowerLimit=0
  MCU2_IdcSensorFaultcv : DataTypeConversion
  MCU2_IuSensorFault_Ad : Sum
  MCU2_IuSensorFault_Convert : DataTypeConversion  OutDataTypeStr=uint32
  MCU2_IuSensorFault_F : Gain
  MCU2_IuSensorFault_L : simulink/Logic and Bit Operations/Bitwise Operator  logicop=AND  UseBitMask=on  BitMask=12  BitMaskRealWorld=Stored Integer
  MCU2_IuSensorFault_O : Constant  Value=0  OutDataTypeStr=single
  MCU2_IuSensorFault_S : ArithShift  BitShiftNumber=2
  MCU2_IuSensorFault_Sub : Subsystem
  MCU2_IuSensorFault_sat : Saturate  UpperLimit=3  LowerLimit=0
  MCU2_IuSensorFaultcv : DataTypeConversion
  MCU2_IvSensorFault_Ad : Sum
  MCU2_IvSensorFault_Convert : DataTypeConversion  OutDataTypeStr=uint32
  MCU2_IvSensorFault_F : Gain
  MCU2_IvSensorFault_L : simulink/Logic and Bit Operations/Bitwise Operator  logicop=AND  UseBitMask=on  BitMask=48  BitMaskRealWorld=Stored Integer
  MCU2_IvSensorFault_O : Constant  Value=0  OutDataTypeStr=single
  MCU2_IvSensorFault_S : ArithShift  BitShiftNumber=4
  MCU2_IvSensorFault_Sub : Subsystem
  MCU2_IvSensorFault_sat : Saturate  UpperLimit=3  LowerLimit=0
  MCU2_IvSensorFaultcv : DataTypeConversion
  MCU2_MemoryFault_Ad : Sum
  MCU2_MemoryFault_Convert : DataTypeConversion  OutDataTypeStr=uint32
  MCU2_MemoryFault_F : Gain
  MCU2_MemoryFault_L : simulink/Logic and Bit Operations/Bitwise Operator  logicop=AND  UseBitMask=on  BitMask=48  BitMaskRealWorld=Stored Integer
  MCU2_MemoryFault_O : Constant  Value=0  OutDataTypeStr=single
  MCU2_MemoryFault_S : ArithShift  BitShiftNumber=4
  MCU2_MemoryFault_Sub : Subsystem
  MCU2_MemoryFault_sat : Saturate  UpperLimit=3  LowerLimit=0
  MCU2_MemoryFaultcv : DataTypeConversion
  MCU2_MotorOverLoad_Ad : Sum
  MCU2_MotorOverLoad_Convert : DataTypeConversion  OutDataTypeStr=uint32
  MCU2_MotorOverLoad_F : Gain
  MCU2_MotorOverLoad_L : simulink/Logic and Bit Operations/Bitwise Operator  logicop=AND  UseBitMask=on  BitMask=3  BitMaskRealWorld=Stored Integer
  MCU2_MotorOverLoad_O : Constant  Value=0  OutDataTypeStr=single
  MCU2_MotorOverLoad_S : ArithShift
  MCU2_MotorOverLoad_Sub : Subsystem
  MCU2_MotorOverLoad_sat : Saturate  UpperLimit=3  LowerLimit=0
  MCU2_MotorOverLoadcv : DataTypeConversion
  MCU2_MotorOverSpeed_Ad : Sum
  MCU2_MotorOverSpeed_Convert : DataTypeConversion  OutDataTypeStr=uint32
  MCU2_MotorOverSpeed_F : Gain
  MCU2_MotorOverSpeed_L : simulink/Logic and Bit Operations/Bitwise Operator  logicop=AND  UseBitMask=on  BitMask=192  BitMaskRealWorld=Stored Integer
  MCU2_MotorOverSpeed_O : Constant  Value=0  OutDataTypeStr=single
  MCU2_MotorOverSpeed_S : ArithShift  BitShiftNumber=6
  MCU2_MotorOverSpeed_Sub : Subsystem
  MCU2_MotorOverSpeed_sat : Saturate  UpperLimit=3  LowerLimit=0
  MCU2_MotorOverSpeedcv : DataTypeConversion
  MCU2_MotorOverTemp_Ad : Sum
  MCU2_MotorOverTemp_Convert : DataTypeConversion  OutDataTypeStr=uint32
  MCU2_MotorOverTemp_F : Gain
  MCU2_MotorOverTemp_L : simulink/Logic and Bit Operations/Bitwise Operator  logicop=AND  UseBitMask=on  BitMask=12  BitMaskRealWorld=Stored Integer
  MCU2_MotorOverTemp_O : Constant  Value=0  OutDataTypeStr=single
  MCU2_MotorOverTemp_S : ArithShift  BitShiftNumber=2
  MCU2_MotorOverTemp_Sub : Subsystem
  MCU2_MotorOverTemp_sat : Saturate  UpperLimit=3  LowerLimit=0
  MCU2_MotorOverTempcv : DataTypeConversion
  MCU2_MotorStallingFault_Ad : Sum
  MCU2_MotorStallingFault_Convert : DataTypeConversion  OutDataTypeStr=uint32
  MCU2_MotorStallingFault_F : Gain
  MCU2_MotorStallingFault_L : simulink/Logic and Bit Operations/Bitwise Operator  logicop=AND  UseBitMask=on  BitMask=12  BitMaskRealWorld=Stored Integer
  MCU2_MotorStallingFault_O : Constant  Value=0  OutDataTypeStr=single
  MCU2_MotorStallingFault_S : ArithShift  BitShiftNumber=2
  MCU2_MotorStallingFault_Sub : Subsystem
  MCU2_MotorStallingFault_sat : Saturate  UpperLimit=3  LowerLimit=0
  MCU2_MotorStallingFaultcv : DataTypeConversion
  MCU2_OverVoltage_Ad : Sum
  MCU2_OverVoltage_Convert : DataTypeConversion  OutDataTypeStr=uint32
  MCU2_OverVoltage_F : Gain
  MCU2_OverVoltage_L : simulink/Logic and Bit Operations/Bitwise Operator  logicop=AND  UseBitMask=on  BitMask=12  BitMaskRealWorld=Stored Integer
  MCU2_OverVoltage_O : Constant  Value=0  OutDataTypeStr=single
  MCU2_OverVoltage_S : ArithShift  BitShiftNumber=2
  MCU2_OverVoltage_Sub : Subsystem
  MCU2_OverVoltage_sat : Saturate  UpperLimit=3  LowerLimit=0
  MCU2_OverVoltagecv : DataTypeConversion
  MCU2_RotaryInverterFault_Ad : Sum
  MCU2_RotaryInverterFault_Convert : DataTypeConversion  OutDataTypeStr=uint32
  MCU2_RotaryInverterFault_F : Gain
  MCU2_RotaryInverterFault_L : simulink/Logic and Bit Operations/Bitwise Operator  logicop=AND  UseBitMask=on  BitMask=192  BitMaskRealWorld=Stored Integer
  MCU2_RotaryInverterFault_O : Constant  Value=0  OutDataTypeStr=single
  MCU2_RotaryInverterFault_S : ArithShift  BitShiftNumber=6
  MCU2_RotaryInverterFault_Sub : Subsystem
  MCU2_RotaryInverterFault_sat : Saturate  UpperLimit=3  LowerLimit=0
  MCU2_RotaryInverterFaultcv : DataTypeConversion
  MCU2_TempSensorFault_Ad : Sum
  MCU2_TempSensorFault_Convert : DataTypeConversion  OutDataTypeStr=uint32
  MCU2_TempSensorFault_F : Gain
  MCU2_TempSensorFault_L : simulink/Logic and Bit Operations/Bitwise Operator  logicop=AND  UseBitMask=on  BitMask=3  BitMaskRealWorld=Stored Integer
  MCU2_TempSensorFault_O : Constant  Value=0  OutDataTypeStr=single
  MCU2_TempSensorFault_S : ArithShift
  MCU2_TempSensorFault_Sub : Subsystem
  MCU2_TempSensorFault_sat : Saturate  UpperLimit=3  LowerLimit=0
  MCU2_TempSensorFaultcv : DataTypeConversion
  MCU2_UdcDetectionFault_Ad : Sum
  MCU2_UdcDetectionFault_Convert : DataTypeConversion  OutDataTypeStr=uint32
  MCU2_UdcDetectionFault_F : Gain
  MCU2_UdcDetectionFault_L : simulink/Logic and Bit Operations/Bitwise Operator  logicop=AND  UseBitMask=on  BitMask=3  BitMaskRealWorld=Stored Integer
  MCU2_UdcDetectionFault_O : Constant  Value=0  OutDataTypeStr=single
  MCU2_UdcDetectionFault_S : ArithShift
  MCU2_UdcDetectionFault_Sub : Subsystem
  MCU2_UdcDetectionFault_sat : Saturate  UpperLimit=3  LowerLimit=0
  MCU2_UdcDetectionFaultcv : DataTypeConversion
  MCU2_UnderVoltage_Ad : Sum
  MCU2_UnderVoltage_Convert : DataTypeConversion  OutDataTypeStr=uint32
  MCU2_UnderVoltage_F : Gain
  MCU2_UnderVoltage_L : simulink/Logic and Bit Operations/Bitwise Operator  logicop=AND  UseBitMask=on  BitMask=48  BitMaskRealWorld=Stored Integer
  MCU2_UnderVoltage_O : Constant  Value=0  OutDataTypeStr=single
  MCU2_UnderVoltage_S : ArithShift  BitShiftNumber=4
  MCU2_UnderVoltage_Sub : Subsystem
  MCU2_UnderVoltage_sat : Saturate  UpperLimit=3  LowerLimit=0
  MCU2_UnderVoltagecv : DataTypeConversion
  MCU2_MotorStallingFault_Out : Outport
  MCU2_UdcDetectionFault_Out : Outport  Port=2
  MCU2_TempSensorFault_Out : Outport  Port=3
  MCU2_ActieDischargingFault_Out : Outport  Port=4
  MCU2_IdcSensorFault_Out : Outport  Port=5
  MCU2_IuSensorFault_Out : Outport  Port=6
  MCU2_IvSensorFault_Out : Outport  Port=7
  MCU2_FaultLevel_Out : Outport  Port=8
  MCU2_ControllerOverload_Out : Outport  Port=9
  MCU2_CanCommunicationFault_Out : Outport  Port=10
  MCU2_MemoryFault_Out : Outport  Port=11
  MCU2_DownratingFault_Out : Outport  Port=12
  MCU2_IGBTFault_Out : Outport  Port=13
  MCU2_MotorOverTemp_Out : Outport  Port=14
  MCU2_ControllerOverTemp_Out : Outport  Port=15
  MCU2_MotorOverSpeed_Out : Outport  Port=16
  MCU2_RotaryInverterFault_Out : Outport  Port=17
  MCU2_UnderVoltage_Out : Outport  Port=18
  MCU2_OverVoltage_Out : Outport  Port=19
  MCU2_MotorOverLoad_Out : Outport  Port=20
  wires:
  MCU2_MotorStallingFault_F/1 -> MCU2_MotorStallingFault_Ad/1
  MCU2_MotorStallingFault_O/1 -> MCU2_MotorStallingFault_Ad/2
  MCU2_MotorStallingFault_Ad/1 -> MCU2_MotorStallingFault_sat/1
  MCU2_MotorStallingFault_sat/1 -> MCU2_MotorStallingFault_Out/1
  Demux/6 -> MCU2_MotorStallingFault_Sub/1(In1), MCU2_UdcDetectionFault_Sub/1(In1)
  MCU2_MotorStallingFault_Sub/1(Out1) -> MCU2_MotorStallingFault_Convert/1
  MCU2_MotorStallingFault_Convert/1 -> MCU2_MotorStallingFault_L/1
  MCU2_MotorStallingFault_L/1 -> MCU2_MotorStallingFault_S/1
  MCU2_MotorStallingFault_S/1 -> MCU2_MotorStallingFaultcv/1
  MCU2_MotorStallingFaultcv/1 -> MCU2_MotorStallingFault_F/1
  MCU2_UdcDetectionFault_F/1 -> MCU2_UdcDetectionFault_Ad/1
  MCU2_UdcDetectionFault_O/1 -> MCU2_UdcDetectionFault_Ad/2
  MCU2_UdcDetectionFault_Ad/1 -> MCU2_UdcDetectionFault_sat/1
  MCU2_UdcDetectionFault_sat/1 -> MCU2_UdcDetectionFault_Out/1
  MCU2_UdcDetectionFault_Sub/1(Out1) -> MCU2_UdcDetectionFault_Convert/1
  MCU2_UdcDetectionFault_Convert/1 -> MCU2_UdcDetectionFault_L/1
  MCU2_UdcDetectionFault_L/1 -> MCU2_UdcDetectionFault_S/1
  MCU2_UdcDetectionFault_S/1 -> MCU2_UdcDetectionFaultcv/1
  MCU2_UdcDetectionFaultcv/1 -> MCU2_UdcDetectionFault_F/1
  MCU2_TempSensorFault_F/1 -> MCU2_TempSensorFault_Ad/1
  MCU2_TempSensorFault_O/1 -> MCU2_TempSensorFault_Ad/2
  MCU2_TempSensorFault_Ad/1 -> MCU2_TempSensorFault_sat/1
  MCU2_TempSensorFault_sat/1 -> MCU2_TempSensorFault_Out/1
  Demux/5 -> MCU2_TempSensorFault_Sub/1(In1), MCU2_ActieDischargingFault_Sub/1(In1)
  MCU2_TempSensorFault_Sub/1(Out1) -> MCU2_TempSensorFault_Convert/1
  MCU2_TempSensorFault_Convert/1 -> MCU2_TempSensorFault_L/1
  MCU2_TempSensorFault_L/1 -> MCU2_TempSensorFault_S/1
  MCU2_TempSensorFault_S/1 -> MCU2_TempSensorFaultcv/1
  MCU2_TempSensorFaultcv/1 -> MCU2_TempSensorFault_F/1
  MCU2_ActieDischargingFault_F/1 -> MCU2_ActieDischargingFault_Ad/1
  MCU2_ActieDischargingFault_O/1 -> MCU2_ActieDischargingFault_Ad/2
  MCU2_ActieDischargingFault_Ad/1 -> MCU2_ActieDischargingFault_sat/1
  MCU2_ActieDischargingFault_sat/1 -> MCU2_ActieDischargingFault_Out/1
  MCU2_ActieDischargingFault_Sub/1(Out1) -> MCU2_ActieDischargingFault_Convert/1
  MCU2_ActieDischargingFault_Convert/1 -> MCU2_ActieDischargingFault_L/1
  MCU2_ActieDischargingFault_L/1 -> MCU2_ActieDischargingFault_S/1
  MCU2_ActieDischargingFault_S/1 -> MCU2_ActieDischargingFaultcv/1
  MCU2_ActieDischargingFaultcv/1 -> MCU2_ActieDischargingFault_F/1
  MCU2_IdcSensorFault_F/1 -> MCU2_IdcSensorFault_Ad/1
  MCU2_IdcSensorFault_O/1 -> MCU2_IdcSensorFault_Ad/2
  MCU2_IdcSensorFault_Ad/1 -> MCU2_IdcSensorFault_sat/1
  MCU2_IdcSensorFault_sat/1 -> MCU2_IdcSensorFault_Out/1
  Demux/4 -> MCU2_IdcSensorFault_Sub/1(In1), MCU2_IuSensorFault_Sub/1(In1), MCU2_IvSensorFault_Sub/1(In1), MCU2_FaultLevel_Sub/1(In1)
  MCU2_IdcSensorFault_Sub/1(Out1) -> MCU2_IdcSensorFault_Convert/1
  MCU2_IdcSensorFault_Convert/1 -> MCU2_IdcSensorFault_L/1
  MCU2_IdcSensorFault_L/1 -> MCU2_IdcSensorFault_S/1
  MCU2_IdcSensorFault_S/1 -> MCU2_IdcSensorFaultcv/1
  MCU2_IdcSensorFaultcv/1 -> MCU2_IdcSensorFault_F/1
  MCU2_IuSensorFault_F/1 -> MCU2_IuSensorFault_Ad/1
  MCU2_IuSensorFault_O/1 -> MCU2_IuSensorFault_Ad/2
  MCU2_IuSensorFault_Ad/1 -> MCU2_IuSensorFault_sat/1
  MCU2_IuSensorFault_sat/1 -> MCU2_IuSensorFault_Out/1
  MCU2_IuSensorFault_Sub/1(Out1) -> MCU2_IuSensorFault_Convert/1
  MCU2_IuSensorFault_Convert/1 -> MCU2_IuSensorFault_L/1
  MCU2_IuSensorFault_L/1 -> MCU2_IuSensorFault_S/1
  MCU2_IuSensorFault_S/1 -> MCU2_IuSensorFaultcv/1
  MCU2_IuSensorFaultcv/1 -> MCU2_IuSensorFault_F/1
  MCU2_IvSensorFault_F/1 -> MCU2_IvSensorFault_Ad/1
  MCU2_IvSensorFault_O/1 -> MCU2_IvSensorFault_Ad/2
  MCU2_IvSensorFault_Ad/1 -> MCU2_IvSensorFault_sat/1
  MCU2_IvSensorFault_sat/1 -> MCU2_IvSensorFault_Out/1
  MCU2_IvSensorFault_Sub/1(Out1) -> MCU2_IvSensorFault_Convert/1
  MCU2_IvSensorFault_Convert/1 -> MCU2_IvSensorFault_L/1
  MCU2_IvSensorFault_L/1 -> MCU2_IvSensorFault_S/1
  MCU2_IvSensorFault_S/1 -> MCU2_IvSensorFaultcv/1
  MCU2_IvSensorFaultcv/1 -> MCU2_IvSensorFault_F/1
  MCU2_FaultLevel_F/1 -> MCU2_FaultLevel_Ad/1
  MCU2_FaultLevel_O/1 -> MCU2_FaultLevel_Ad/2
  MCU2_FaultLevel_Ad/1 -> MCU2_FaultLevel_sat/1
  MCU2_FaultLevel_sat/1 -> MCU2_FaultLevel_Out/1
  MCU2_FaultLevel_Sub/1(Out1) -> MCU2_FaultLevel_Convert/1
  MCU2_FaultLevel_Convert/1 -> MCU2_FaultLevel_L/1
  MCU2_FaultLevel_L/1 -> MCU2_FaultLevel_S/1
  MCU2_FaultLevel_S/1 -> MCU2_FaultLevelcv/1
  MCU2_FaultLevelcv/1 -> MCU2_FaultLevel_F/1
  MCU2_ControllerOverload_F/1 -> MCU2_ControllerOverload_Ad/1
  MCU2_ControllerOverload_O/1 -> MCU2_ControllerOverload_Ad/2
  MCU2_ControllerOverload_Ad/1 -> MCU2_ControllerOverload_sat/1
  MCU2_ControllerOverload_sat/1 -> MCU2_ControllerOverload_Out/1
  Demux/1 -> MCU2_UnderVoltage_Sub/1(In1), MCU2_OverVoltage_Sub/1(In1), MCU2_ControllerOverload_Sub/1(In1), MCU2_RotaryInverterFault_Sub/1(In1)
  MCU2_ControllerOverload_Sub/1(Out1) -> MCU2_ControllerOverload_Convert/1
  MCU2_ControllerOverload_Convert/1 -> MCU2_ControllerOverload_L/1
  MCU2_ControllerOverload_L/1 -> MCU2_ControllerOverload_S/1
  MCU2_ControllerOverload_S/1 -> MCU2_ControllerOverloadcv/1
  MCU2_ControllerOverloadcv/1 -> MCU2_ControllerOverload_F/1
  MCU2_CanCommunicationFault_F/1 -> MCU2_CanCommunicationFault_Ad/1
  MCU2_CanCommunicationFault_O/1 -> MCU2_CanCommunicationFault_Ad/2
  MCU2_CanCommunicationFault_Ad/1 -> MCU2_CanCommunicationFault_sat/1
  MCU2_CanCommunicationFault_sat/1 -> MCU2_CanCommunicationFault_Out/1
  Demux/3 -> MCU2_DownratingFault_Sub/1(In1), MCU2_MotorOverLoad_Sub/1(In1), MCU2_MemoryFault_Sub/1(In1), MCU2_CanCommunicationFault_Sub/1(In1)
  MCU2_CanCommunicationFault_Sub/1(Out1) -> MCU2_CanCommunicationFault_Convert/1
  MCU2_CanCommunicationFault_Convert/1 -> MCU2_CanCommunicationFault_L/1
  MCU2_CanCommunicationFault_L/1 -> MCU2_CanCommunicationFault_S/1
  MCU2_CanCommunicationFault_S/1 -> MCU2_CanCommunicationFaultcv/1
  MCU2_CanCommunicationFaultcv/1 -> MCU2_CanCommunicationFault_F/1
  MCU2_MemoryFault_F/1 -> MCU2_MemoryFault_Ad/1
  MCU2_MemoryFault_O/1 -> MCU2_MemoryFault_Ad/2
  MCU2_MemoryFault_Ad/1 -> MCU2_MemoryFault_sat/1
  MCU2_MemoryFault_sat/1 -> MCU2_MemoryFault_Out/1
  MCU2_MemoryFault_Sub/1(Out1) -> MCU2_MemoryFault_Convert/1
  MCU2_MemoryFault_Convert/1 -> MCU2_MemoryFault_L/1
  MCU2_MemoryFault_L/1 -> MCU2_MemoryFault_S/1
  MCU2_MemoryFault_S/1 -> MCU2_MemoryFaultcv/1
  MCU2_MemoryFaultcv/1 -> MCU2_MemoryFault_F/1
  MCU2_DownratingFault_F/1 -> MCU2_DownratingFault_Ad/1
  MCU2_DownratingFault_O/1 -> MCU2_DownratingFault_Ad/2
  MCU2_DownratingFault_Ad/1 -> MCU2_DownratingFault_sat/1
  MCU2_DownratingFault_sat/1 -> MCU2_DownratingFault_Out/1
  MCU2_DownratingFault_Sub/1(Out1) -> MCU2_DownratingFault_Convert/1
  MCU2_DownratingFault_Convert/1 -> MCU2_DownratingFault_L/1
  MCU2_DownratingFault_L/1 -> MCU2_DownratingFault_S/1
  MCU2_DownratingFault_S/1 -> MCU2_DownratingFaultcv/1
  MCU2_DownratingFaultcv/1 -> MCU2_DownratingFault_F/1
  MCU2_IGBTFault_F/1 -> MCU2_IGBTFault_Ad/1
  MCU2_IGBTFault_O/1 -> MCU2_IGBTFault_Ad/2
  MCU2_IGBTFault_Ad/1 -> MCU2_IGBTFault_sat/1
  MCU2_IGBTFault_sat/1 -> MCU2_IGBTFault_Out/1
  Demux/2 -> MCU2_ControllerOverTemp_Sub/1(In1), MCU2_MotorOverSpeed_Sub/1(In1), MCU2_IGBTFault_Sub/1(In1), MCU2_MotorOverTemp_Sub/1(In1)
  MCU2_IGBTFault_Sub/1(Out1) -> MCU2_IGBTFault_Convert/1
  MCU2_IGBTFault_Convert/1 -> MCU2_IGBTFault_L/1
  MCU2_IGBTFault_L/1 -> MCU2_IGBTFault_S/1
  MCU2_IGBTFault_S/1 -> MCU2_IGBTFaultcv/1
  MCU2_IGBTFaultcv/1 -> MCU2_IGBTFault_F/1
  MCU2_MotorOverTemp_F/1 -> MCU2_MotorOverTemp_Ad/1
  MCU2_MotorOverTemp_O/1 -> MCU2_MotorOverTemp_Ad/2
  MCU2_MotorOverTemp_Ad/1 -> MCU2_MotorOverTemp_sat/1
  MCU2_MotorOverTemp_sat/1 -> MCU2_MotorOverTemp_Out/1
  MCU2_MotorOverTemp_Sub/1(Out1) -> MCU2_MotorOverTemp_Convert/1
  MCU2_MotorOverTemp_Convert/1 -> MCU2_MotorOverTemp_L/1
  MCU2_MotorOverTemp_L/1 -> MCU2_MotorOverTemp_S/1
  MCU2_MotorOverTemp_S/1 -> MCU2_MotorOverTempcv/1
  MCU2_MotorOverTempcv/1 -> MCU2_MotorOverTemp_F/1
  MCU2_ControllerOverTemp_F/1 -> MCU2_ControllerOverTemp_Ad/1
  MCU2_ControllerOverTemp_O/1 -> MCU2_ControllerOverTemp_Ad/2
  MCU2_ControllerOverTemp_Ad/1 -> MCU2_ControllerOverTemp_sat/1
  MCU2_ControllerOverTemp_sat/1 -> MCU2_ControllerOverTemp_Out/1
  MCU2_ControllerOverTemp_Sub/1(Out1) -> MCU2_ControllerOverTemp_Convert/1
  MCU2_ControllerOverTemp_Convert/1 -> MCU2_ControllerOverTemp_L/1
  MCU2_ControllerOverTemp_L/1 -> MCU2_ControllerOverTemp_S/1
  MCU2_ControllerOverTemp_S/1 -> MCU2_ControllerOverTempcv/1
  MCU2_ControllerOverTempcv/1 -> MCU2_ControllerOverTemp_F/1
  MCU2_MotorOverSpeed_F/1 -> MCU2_MotorOverSpeed_Ad/1
  MCU2_MotorOverSpeed_O/1 -> MCU2_MotorOverSpeed_Ad/2
  MCU2_MotorOverSpeed_Ad/1 -> MCU2_MotorOverSpeed_sat/1
  MCU2_MotorOverSpeed_sat/1 -> MCU2_MotorOverSpeed_Out/1
  MCU2_MotorOverSpeed_Sub/1(Out1) -> MCU2_MotorOverSpeed_Convert/1
  MCU2_MotorOverSpeed_Convert/1 -> MCU2_MotorOverSpeed_L/1
  MCU2_MotorOverSpeed_L/1 -> MCU2_MotorOverSpeed_S/1
  MCU2_MotorOverSpeed_S/1 -> MCU2_MotorOverSpeedcv/1
  MCU2_MotorOverSpeedcv/1 -> MCU2_MotorOverSpeed_F/1
  MCU2_RotaryInverterFault_F/1 -> MCU2_RotaryInverterFault_Ad/1
  MCU2_RotaryInverterFault_O/1 -> MCU2_RotaryInverterFault_Ad/2
  MCU2_RotaryInverterFault_Ad/1 -> MCU2_RotaryInverterFault_sat/1
  MCU2_RotaryInverterFault_sat/1 -> MCU2_RotaryInverterFault_Out/1
  MCU2_RotaryInverterFault_Sub/1(Out1) -> MCU2_RotaryInverterFault_Convert/1
  MCU2_RotaryInverterFault_Convert/1 -> MCU2_RotaryInverterFault_L/1
  MCU2_RotaryInverterFault_L/1 -> MCU2_RotaryInverterFault_S/1
  MCU2_RotaryInverterFault_S/1 -> MCU2_RotaryInverterFaultcv/1
  MCU2_RotaryInverterFaultcv/1 -> MCU2_RotaryInverterFault_F/1
  MCU2_UnderVoltage_F/1 -> MCU2_UnderVoltage_Ad/1
  MCU2_UnderVoltage_O/1 -> MCU2_UnderVoltage_Ad/2
  MCU2_UnderVoltage_Ad/1 -> MCU2_UnderVoltage_sat/1
  MCU2_UnderVoltage_sat/1 -> MCU2_UnderVoltage_Out/1
  MCU2_UnderVoltage_Sub/1(Out1) -> MCU2_UnderVoltage_Convert/1
  MCU2_UnderVoltage_Convert/1 -> MCU2_UnderVoltage_L/1
  MCU2_UnderVoltage_L/1 -> MCU2_UnderVoltage_S/1
  MCU2_UnderVoltage_S/1 -> MCU2_UnderVoltagecv/1
  MCU2_UnderVoltagecv/1 -> MCU2_UnderVoltage_F/1
  MCU2_OverVoltage_F/1 -> MCU2_OverVoltage_Ad/1
  MCU2_OverVoltage_O/1 -> MCU2_OverVoltage_Ad/2
  MCU2_OverVoltage_Ad/1 -> MCU2_OverVoltage_sat/1
  MCU2_OverVoltage_sat/1 -> MCU2_OverVoltage_Out/1
  MCU2_OverVoltage_Sub/1(Out1) -> MCU2_OverVoltage_Convert/1
  MCU2_OverVoltage_Convert/1 -> MCU2_OverVoltage_L/1
  MCU2_OverVoltage_L/1 -> MCU2_OverVoltage_S/1
  MCU2_OverVoltage_S/1 -> MCU2_OverVoltagecv/1
  MCU2_OverVoltagecv/1 -> MCU2_OverVoltage_F/1
  MCU2_MotorOverLoad_F/1 -> MCU2_MotorOverLoad_Ad/1
  MCU2_MotorOverLoad_O/1 -> MCU2_MotorOverLoad_Ad/2
  MCU2_MotorOverLoad_Ad/1 -> MCU2_MotorOverLoad_sat/1
  MCU2_MotorOverLoad_sat/1 -> MCU2_MotorOverLoad_Out/1
  MCU2_MotorOverLoad_Sub/1(Out1) -> MCU2_MotorOverLoad_Convert/1
  MCU2_MotorOverLoad_Convert/1 -> MCU2_MotorOverLoad_L/1
  MCU2_MotorOverLoad_L/1 -> MCU2_MotorOverLoad_S/1
  MCU2_MotorOverLoad_S/1 -> MCU2_MotorOverLoadcv/1
  MCU2_MotorOverLoadcv/1 -> MCU2_MotorOverLoad_F/1
  input/1 -> Demux/1
